simulink library "output_prep_lib"  (R2016b)
settings: Solver=ode45  StartTime=0.0  StopTime=10.0  RelTol=1e-3  EnableMultiTasking=on
undefined symbols (not defined in the file): ase_status_acquiring, ase_status_converged, ase_status_diverged, ase_total_num_states, confidence, cov_diag, tun_abp_p_imu_body_body, tun_ase_acquired_ticks, tun_ase_converged_thresh, tun_ase_diverged_thresh
libraries: simulink x9, math_utils x1
settings Model: Creator=jfusco1  LastModifiedBy=jfusco1
settings DataIOCC: LimitDataPoints=on  SaveFormat=Array
settings OptimizationCC: LifeSpan=inf
settings DebuggingCC: AllowSymbolicDim=off  SFUnexpectedBacktrackingDiag=warning  SFNoUnconditionalDefaultTransitionDiag=warning  SFExecutionAtInitializationDiag=none
settings HardwareCC: ProdBitPerPointer=32  ProdBitPerSizeT=32  ProdBitPerPtrDiffT=32  ProdLargestAtomicFloat=None  ProdIntDivRoundTo=Undefined  ProdEndianess=Unspecified  ProdWordSize=32  ProdHWDeviceType=32-bit Generic
settings ModelReferenceCC: PropagateSignalLabelsOutOfModel=off
settings GRTTargetCC: TargetLangStandard=C89/C90 (ANSI)  GeneratePreprocessorConditionals=Disable all
settings ConfigComp: CovMetricSettings=dw  CovHtmlReporting=on  CovSaveCumulativeToWorkspaceVar=on  CovSaveSingleToWorkspaceVar=on  CovExternalEMLEnable=off

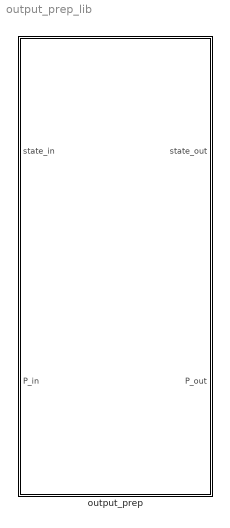
== system output_prep_lib ==
  output_prep : Subsystem

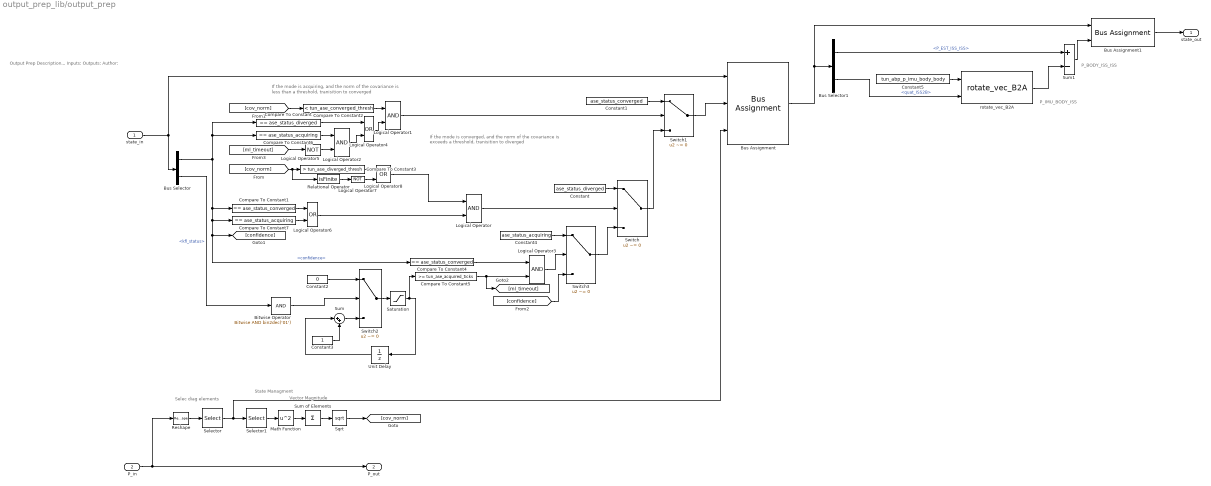
== system output_prep_lib/output_prep ==
  note: P_BODY_ISS_ISS
  note: If the mode is converged, and the norm of the covariance
      | is exceeds a threshold, tranisition to diverged
  note: If the mode is acquiring, and the norm of the covariance
      | is less than a threshold, tranisition to converged
  note: Vector Magnitude
  note: Selec diag elements
  note: Output Prep
      | Description...
      |
      | Inputs:
      |
      | Outputs:
      |
      | Author:
  note: State Managment
  note: P_IMU_BODY_ISS
  state_in : Inport  OutDataTypeStr=Bus: kfl_msg
  P_in : Inport  Port=2  OutDataTypeStr=ase_cov_datatype
  Bitwise Operator : simulink/Logic and Bit Operations/Bitwise Operator  logicop=AND  UseBitMask=on  BitMask=bin2dec('01')  BitMaskRealWorld=Stored Integer
  Bus Assignment : BusAssignment  AssignedSignals=confidence,cov_diag
  Bus Assignment1 : BusAssignment  AssignedSignals=P_B_ISS_ISS
  Bus Selector : BusSelector  OutputSignals=confidence,kfl_status
  Bus Selector1 : BusSelector  OutputSignals=P_EST_ISS_ISS,quat_ISS2B
  Compare To Constant : simulink/Logic and Bit Operations/Compare To Constant  relop===  const=ase_status_diverged  OutDataTypeStr=boolean
  Compare To Constant1 : simulink/Logic and Bit Operations/Compare To Constant  relop===  const=ase_status_converged  OutDataTypeStr=boolean
  Compare To Constant2 : simulink/Logic and Bit Operations/Compare To Constant  relop=<  const=tun_ase_converged_thresh  OutDataTypeStr=boolean
  Compare To Constant3 : simulink/Logic and Bit Operations/Compare To Constant  relop=>  const=tun_ase_diverged_thresh  OutDataTypeStr=boolean
  Compare To Constant4 : simulink/Logic and Bit Operations/Compare To Constant  relop===  const=ase_status_converged  OutDataTypeStr=boolean
  Compare To Constant5 : simulink/Logic and Bit Operations/Compare To Constant  relop=>=  const=tun_ase_acquired_ticks  OutDataTypeStr=boolean
  Compare To Constant6 : simulink/Logic and Bit Operations/Compare To Constant  relop===  const=ase_status_acquiring  OutDataTypeStr=boolean
  Compare To Constant7 : simulink/Logic and Bit Operations/Compare To Constant  relop===  const=ase_status_acquiring  OutDataTypeStr=boolean
  Constant : Constant  Value=ase_status_diverged
  Constant1 : Constant  Value=ase_status_converged
  Constant2 : Constant  Value=0
  Constant3 : Constant
  Constant4 : Constant  Value=ase_status_acquiring
  Constant5 : Constant  Value=tun_abp_p_imu_body_body
  Logical Operator{,1..3} (4 alike) : Logic  AllPortsSameDT=off  OutDataTypeStr=boolean
  Logical Operator4 : Logic  Operator=OR  AllPortsSameDT=off  OutDataTypeStr=boolean
  Logical Operator5 : Logic  Operator=NOT  AllPortsSameDT=off  OutDataTypeStr=boolean
  Logical Operator6 : Logic  Operator=OR  AllPortsSameDT=off  OutDataTypeStr=boolean
  Logical Operator7 : Logic  Operator=NOT  Inputs=1  AllPortsSameDT=off  OutDataTypeStr=boolean
  Logical Operator8 : Logic  Operator=OR  AllPortsSameDT=off  OutDataTypeStr=boolean
  Math Function : Math  Operator=square  SaturateOnIntegerOverflow=on
  Relational Operator : RelationalOperator  Operator=isFinite  OutDataTypeStr=boolean  RndMeth=Nearest
  Reshape : Reshape  OutputDimensions=[21*21]
  Saturation : Saturate  UpperLimit=tun_ase_acquired_ticks  LowerLimit=0
  Selector : Selector  InputPortWidth=ase_total_num_states^2  IndexOptions=Index vector (dialog)  Indices=ase_diag_indx  OutputSizes=1
  Selector1 : Selector  InputPortWidth=ase_total_num_states  IndexOptions=Index vector (dialog)  Indices=13:15  OutputSizes=1
  Sqrt : Sqrt  SaturateOnIntegerOverflow=on
  Sum : Sum  Inputs=|++
  Sum of Elements : Sum  Inputs=+
  Sum1 : Sum  Inputs=+-
  Switch{,1..3} (4 alike) : Switch  Criteria=u2 ~= 0
  Unit Delay : UnitDelay  SampleTime=-1
  rotate_vec_B2A : math_utils/rotate_vec_B2A  SystemSampleTime=-1
  state_out : Outport  OutDataTypeStr=Bus: kfl_msg
  P_out : Outport  Port=2
  wires:
  rotate_vec_B2A/1 -> Sum1/2
  Constant5/1 -> rotate_vec_B2A/1
  Bus Selector1/2 -> rotate_vec_B2A/2  "<quat_ISS2B>"
  Sum1/1 -> Bus Assignment1/2
  Bus Selector1/1 -> Sum1/1  "<P_EST_ISS_ISS>"
  Bus Assignment1/1 -> state_out/1
  Selector/1 -> Selector1/1, Bus Assignment/3
  Switch1/1 -> Bus Assignment/2
  Bus Assignment/1 -> Bus Selector1/1, Bus Assignment1/1
  Constant1/1 -> Switch1/1
  Constant/1 -> Switch/1
  Switch/1 -> Switch1/3
  Logical Operator1/1 -> Switch1/2
  Compare To Constant2/1 -> Logical Operator1/1
  [cov_norm] -> Compare To Constant2/1
  Logical Operator/1 -> Switch/2
  Logical Operator6/1 -> Logical Operator/2
  [cov_norm] -> Relational Operator/1, Compare To Constant3/1
  Sqrt/1 -> [cov_norm]
  Bus Selector/1 -> Compare To Constant6/1, Compare To Constant/1, Compare To Constant7/1, Compare To Constant4/1, [confidence], Compare To Constant1/1  "<confidence>"
  state_in/1 -> Bus Assignment/1, Bus Selector/1
  Sum of Elements/1 -> Sqrt/1
  Math Function/1 -> Sum of Elements/1
  Reshape/1 -> Selector/1
  P_in/1 -> Reshape/1, P_out/1
  Selector1/1 -> Math Function/1
  Bus Selector/2 -> Bitwise Operator/1  "<kfl_status>"
  Constant2/1 -> Switch2/1
  Bitwise Operator/1 -> Switch2/2
  Switch2/1 -> Saturation/1
  Unit Delay/1 -> Sum/1
  Sum/1 -> Switch2/3
  Constant3/1 -> Sum/2
  Saturation/1 -> Compare To Constant5/1, Unit Delay/1
  Compare To Constant4/1 -> Logical Operator3/1
  Compare To Constant5/1 -> [ml_timeout], Logical Operator3/2
  Constant4/1 -> Switch3/1
  Logical Operator3/1 -> Switch3/2
  Switch3/1 -> Switch/3
  [confidence] -> Switch3/3
  Logical Operator4/1 -> Logical Operator1/2
  Compare To Constant/1 -> Logical Operator4/1
  [ml_timeout] -> Logical Operator5/1
  Logical Operator2/1 -> Logical Operator4/2
  Compare To Constant6/1 -> Logical Operator2/1
  Logical Operator5/1 -> Logical Operator2/2
  Compare To Constant1/1 -> Logical Operator6/1
  Compare To Constant7/1 -> Logical Operator6/2
  Relational Operator/1 -> Logical Operator7/1
  Compare To Constant3/1 -> Logical Operator8/1
  Logical Operator7/1 -> Logical Operator8/2
  Logical Operator8/1 -> Logical Operator/1
